simulink model "Pouziti_Dashboard"  (R2020b)
settings: Solver=VariableStepAuto  StartTime=0.0  StopTime=2000  MaxStep=0.001  RelTol=1e-3  EnableMultiTasking=on
PreLoadFcn:
  | A1 = 0.2;
  | A01 = 0.001;
  | 
  | A2 = 0.2;
  | A02 = 0.001;
  | 
  | g = 9.81;
CloseFcn:
  | clear A01 A02 A1 A2 g
settings Model: Creator=Jirkovsk  LastModifiedBy=jirkovsky
settings DataIOCC: ReturnWorkspaceOutputs=off
settings OptimizationCC: LifeSpan=inf
settings DebuggingCC: SFUnexpectedBacktrackingDiag=warning  SFNoUnconditionalDefaultTransitionDiag=warning  SFExecutionAtInitializationDiag=none  ArithmeticOperatorsInVariantConditions=warning
settings SFSimCC: SimUseLocalCustomCode=off  CustomCodeUndefinedFunction=UseInterfaceOnly
settings RTWCC: RTWUseLocalCustomCode=off
settings CodeAppCC: StateflowObjectComments=on
settings GRTTargetCC: TargetLangStandard=C89/C90 (ANSI)
settings ConfigComp: CovMetricSettings=dw  CovSaveCumulativeToWorkspaceVar=on  CovSaveSingleToWorkspaceVar=on  CovExternalEMLEnable=off

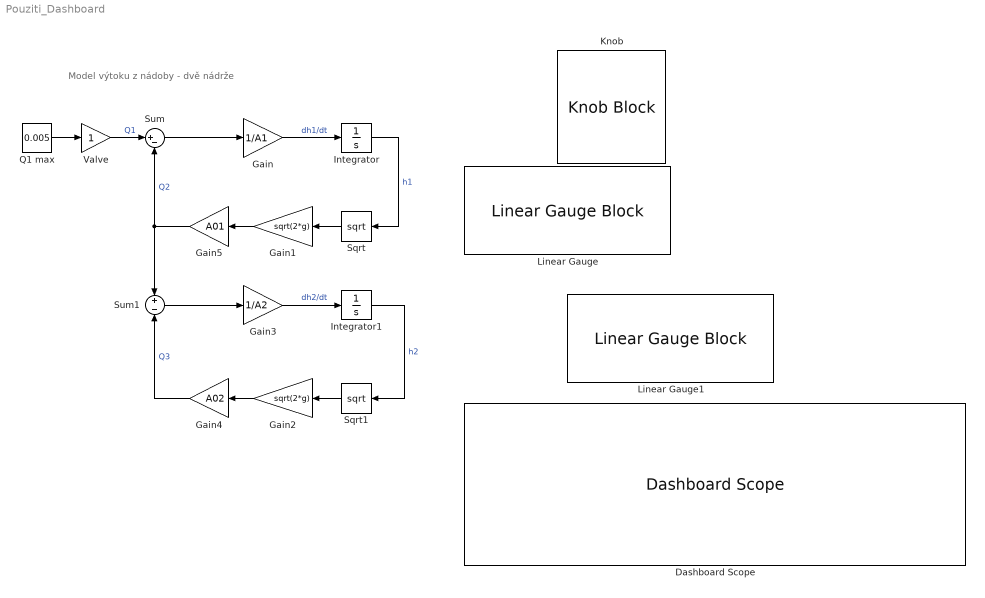
== system Pouziti_Dashboard ==
  note: Model výtoku z nádoby - dvě nádrže
  Dashboard Scope : DashboardScope  Ymin=0  Ymax=2  ScaleAtStop=off
  Gain : Gain  Gain=1/A1
  Gain1 : Gain  Gain=sqrt(2*g)
  Gain2 : Gain  Gain=sqrt(2*g)
  Gain3 : Gain  Gain=1/A2
  Gain4 : Gain  Gain=A02
  Gain5 : Gain  Gain=A01
  Integrator : Integrator  LimitOutput=on  LowerSaturationLimit=0
  Integrator1 : Integrator  LimitOutput=on  LowerSaturationLimit=0
  Knob : KnobBlock  ScaleMax=1
  Linear Gauge : LinearGaugeBlock  ScaleMax=1.5  TickInterval=0.5
  Linear Gauge1 : LinearGaugeBlock  ScaleMax=1.5  TickInterval=0.5
  Q1 max : Constant  Value=0.005
  Sqrt : Sqrt  SaturateOnIntegerOverflow=on
  Sqrt1 : Sqrt  SaturateOnIntegerOverflow=on
  Sum : Sum  Inputs=|+-
  Sum1 : Sum  Inputs=+-
  Valve : Gain
  wires:
  Gain/1 -> Integrator/1  "dh1/dt"
  Q1 max/1 -> Valve/1
  Integrator/1 -> Sqrt/1  "h1"
  Sqrt/1 -> Gain1/1
  Gain1/1 -> Gain5/1
  Sum1/1 -> Gain3/1
  Integrator1/1 -> Sqrt1/1  "h2"
  Sqrt1/1 -> Gain2/1
  Gain4/1 -> Sum1/2  "Q3"
  Sum/1 -> Gain/1
  Gain3/1 -> Integrator1/1  "dh2/dt"
  Gain2/1 -> Gain4/1
  Gain5/1 -> Sum/2, Sum1/1  "Q2"
  Valve/1 -> Sum/1  "Q1"
